simulink model "simulink_model_traverse"  (R2021b)
settings: Solver=ode45  StartTime=0.0  StopTime=20  RelTol=1e-3
model workspace (MAT data in the model file):
  real_gyro_traverse_system = frd
  real_gyro_traverse_system.IOSize_ = [1 1]
  real_gyro_traverse_system.Data_ = ltipack.frddata
  real_gyro_traverse_system.Data_.Frequency = [6.28310441366 6.33210341522 6.38148441394 6.43125040589 6.48140513613 6.53195010269 6.58288979967 6.63422647409 6.68596387104 6.73810423754 6.7906520677 6.84360885953 ... (801 elements, 801x1)]
  real_gyro_traverse_system.Data_.Response = [0.0415989533067-0.25452619791i 0.0397742167115-0.252204239368i 0.0379806235433-0.249895423651i 0.0362177714705-0.247599869967i 0.0344851389527-0.245317786932i 0.0297197960317-0.238508492708i 0.0252005718648-0.231830269098i 0.0209181196988-0.225282818079i 0.0168635360897-0.218866020441i 0.0203672014177-0.220373362303i 0.0239223502576-0.221838980913i 0.0275287441909-0.223261684179i ... (801 elements, 1x1x801)]
  real_gyro_traverse_system.Data_.Delay.Input = 0
  real_gyro_traverse_system.Data_.Delay.Output = 0
  real_gyro_traverse_system.Data_.Delay.IO = 0
  real_gyro_traverse_system.Data_.Ts = 0
  real_gyro_traverse_system.FrequencyUnit_ = 'Hz'
values from neighbouring files (symbols this model uses):
  fric_gear_motor_traverse = 0.021    [loading_project.m]
  fric_gear_turrent_gun_traverse = 1.272    [loading_project.m]
  ts3 = 10^-3    (= 0.001)    [loading_project.m]
libraries: simulink x3, dspsrcs4 x1
(part 1 of 2)
settings Model: Creator=itama  LastModifiedBy=noait

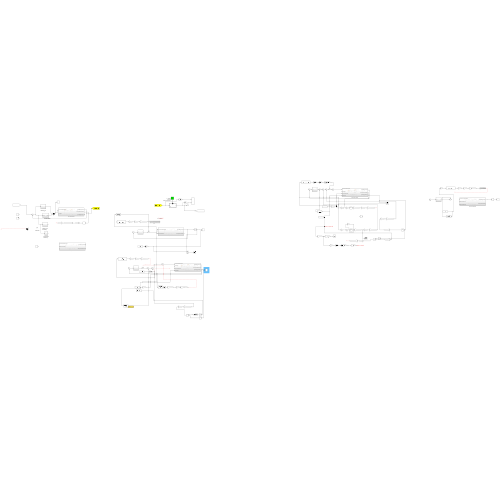
[thumbnail: Simulink's stored preview of the top-level diagram]
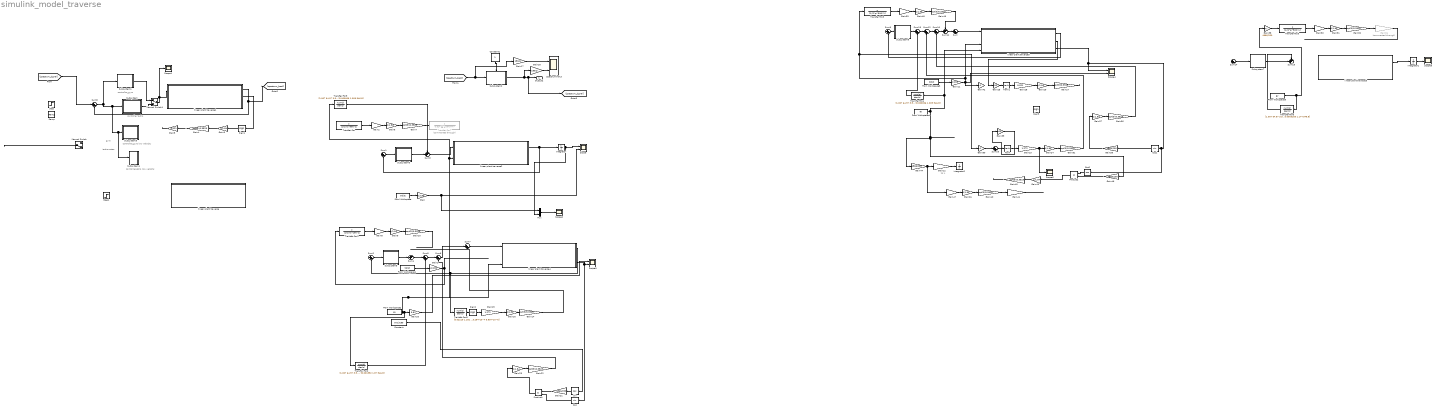
== system simulink_model_traverse ==
  note: controller_gyro
  note: gyro
  note: tachometer
  note: controller tacho
  note: controller_gyro
      | low velocity
  note: controller_taho
      | low velocity
  note: 1/J L
  note: 1/J L
  Constant : Constant  Value=0*pi/180  SampleTime=-1
  Constant1 : Constant  OutDataTypeStr=boolean
      settings: AttributesFormatString=1 - START\n0 -STOP\ninternal spectrum
      settings: OpenFcn=|
      | if get_param(gcbh,'value')-48 set_param(gcbh,'value','0','backgroundcolor','red');
      | else set_param(gcbh,'value','1','backgroundcolor','green');
      | end
  Cos : Trigonometry
  Cos1 : Trigonometry
  Cos2 : Trigonometry  Operator=cos
  From Workspace : FromWorkspace  VariableName=trdist  SampleTime=ts3/3  ZeroCross=off  OutputAfterFinalValue=Setting to zero
  From Workspace1 : FromWorkspace  VariableName=trdist  SampleTime=ts3/3  ZeroCross=off  OutputAfterFinalValue=Setting to zero
  From Workspace2 : FromWorkspace  VariableName=gy  SampleTime=ts3/3  Interpolate=off  ZeroCross=off  OutputAfterFinalValue=Setting to zero
  From Workspace3 : FromWorkspace  VariableName=trdist  SampleTime=ts3/3  Interpolate=off  ZeroCross=off  OutputAfterFinalValue=Setting to zero
  From Workspace4 : FromWorkspace  VariableName=gy  SampleTime=ts3/3  Interpolate=off  ZeroCross=off  OutputAfterFinalValue=Setting to zero
  From Workspace5 : FromWorkspace  VariableName=gy  SampleTime=ts3/3  Interpolate=off  ZeroCross=off  OutputAfterFinalValue=Setting to zero
  Gain : Gain  Gain=pi/180
  Gain1 : Gain  Gain=pi/180
  Gain{4,7,10,14,22,27,32,36,40,45,49,51} (12 alike) : Gain  Gain=sqrt(3)/0.3525
  Gain11 : Gain  Gain=pi/180
  Gain12 : Gain  Gain=-1/0.2189801
  Gain13 : Gain  Gain=1.272
  Gain15 : Gain  Gain=1.272
  Gain{3,6,9,16,23..24,26,29,31,37,43,48} (12 alike) : Gain  Gain=1/1.84
  Gain17 : Gain  Gain=180/pi
  Gain18 : Gain  Gain=180/pi
  Gain{2,8,30,33,47} (5 alike) : Gain  Gain=0.0093
  Gain20 : Gain  Gain=9.81
  Gain{21,35,38,44,46} (5 alike) : Gain  Gain=4866/200
  Gain25 : Gain  Gain=100
  Gain28 : Gain  Gain=0.021
  Gain34 : Gain  Commented=through  Gain=1/0.2189801
  Gain39 : Gain  Gain=100
  Gain41 : Gain  Gain=1/0.2189801
  Gain42 : Gain  Gain=-1
  Gain5 : Gain  Gain=0.021
  Gain50 : Gain  Gain=-1
  Integrator : Integrator
  Integrator1 : Integrator
  Integrator2 : Integrator  ZeroCross=off
  Manual Switch : ManualSwitch  CurrentSetting=0
  Manual Switch1 : ManualSwitch
  Mux : Mux  Inputs=2
  Product1 : Product
  Product2 : Product
  Ramp : simulink/Sources/Ramp  slope=1  start=0  InitialOutput=0
  Scope : Scope  NumInputPorts=2
  Scope{1..2,5..6} (4 alike) : Scope
  Scope3 : Scope  NumInputPorts=2
  Scope4 : Scope  NumInputPorts=2
  Sign1 : Signum
  Sign2 : Signum
  Sign3 : Signum  ZeroCross=off
  Sin : Trigonometry  Operator=cos
  SpectrumInOut : Scope  NumInputPorts=2
  Step : Step  After=0.05  SampleTime=0
  Step1 : Step  After=10*pi/180  SampleTime=0
  Subsystem : Subsystem
  Subsystem1 : Subsystem
  Subsystem2 : Subsystem  mask{GAIN=1%2*pi/180%0.5*pi/180, InitFreq=1, TargetTime=500, FreqAtTime=500}
      mask prompts: InitFreq "INITIAL FREQUENCY"; TargetTime "Target Time"; FreqAtTime "Frequency at Time"
  Subsystem3 : Subsystem
  Subsystem4 : Subsystem
  Subsystem5 : Subsystem
  Subsystem6 : Subsystem
  Subsystem7 : Subsystem
  Subsystem8 : Subsystem
  Sum{,5,7,12..13,16} (6 alike) : Sum  Inputs=|++
  Sum{1..2,6,8..10,14} (7 alike) : Sum  Inputs=|+-
  Sum11 : Sum  Inputs=-+|
  Sum15 : Sum  Inputs=++|
  Sum3 : Sum  Inputs=++|
  Sum4 : Sum  Inputs=-+|
  Tanh : Trigonometry  Operator=tanh
  Tanh1 : Trigonometry  Operator=tanh
  Transfer Fcn : TransferFcn  Numerator=[1 0]  Denominator=[1/(2*pi*500) 1]
  Transfer Fcn1 : TransferFcn  Numerator=[1 0]  Denominator=[1/(2*pi*100) 1]
  Transfer Fcn2 : TransferFcn  Numerator=[1.007 64.97 3.552*10^4]  Denominator=[0.001592 1.87 546.8]
  Transfer Fcn3 : TransferFcn  Numerator=[1 0]  Denominator=[1/(2*pi*500) 1]
  Transfer Fcn4 : TransferFcn  Numerator=[1.007 64.97 3.552*10^4]  Denominator=[0.000006 1.009 546.8]
  Transfer Fcn5 : TransferFcn  Numerator=[1 0]  Denominator=[1/(2*pi*500) 1]
  Transfer Fcn6 : TransferFcn  Numerator=[1.007 64.97 3.552*10^4]  Denominator=[0.0003183 1.174 546.8]
  Transfer Fcn7 : TransferFcn  Commented=through  Numerator=[1 0]  Denominator=[0.6 328.0575777]
  Transfer Fcn8 : TransferFcn  Numerator=[0.02219 1.182 1026 1.42*10^4 5.857*10^6]  Denominator="[0.003183 2.538  528.2 3.284*10^4 5.857*10^6]"
  Transfer Fcn9 : TransferFcn  Numerator=[1.007 64.97 3.552*10^4]  Denominator=[0.000006 1.009 546.8]
  linear plant traverse : Subsystem
  linear plant traverse1 : Subsystem
  linear plant traverse2 : Subsystem
  linear plant traverse3 : Subsystem
  linear plant traverse4 : Subsystem
  linear plant traverse5 : Subsystem
  Output2 : Outport
  wires:
  Manual Switch/1 -> ?
  Subsystem/1(Out1) -> Manual Switch1/2
  Constant1/1 -> Subsystem2/Enable
  Subsystem2/1(Output2) -> [spectrum_signal], Output2/1, Gain18/1
  Gain18/1 -> SpectrumInOut/2
  [spectrum_back] -> Gain17/1, Subsystem2/1(Input)
  Gain17/1 -> SpectrumInOut/1
  Sum8/1 -> Subsystem1/1(In1), Subsystem4/1(In1), Subsystem3/1(In1), Subsystem/1(In1)
  Manual Switch1/1 -> Scope1/1, linear plant traverse1/1(current command traverse)
  linear plant traverse1/2(motor speed tachometer) -> Sign1/1
  Gain4/1 -> Gain5/1
  Gain3/1 -> Gain4/1
  Sign1/1 -> Gain3/1
  Subsystem1/1(Output) -> Manual Switch1/1
  Gain5/1 -> ?
  linear plant traverse1/1(gun speed gyroscope) -> [spectrum_back], Sum8/2
  Sum1/1 -> Subsystem6/1(In1)
  linear plant traverse2/1(gun speed gyroscope) -> Integrator/1, Sum1/2
  From Workspace/1 -> Gain/1
  Gain/1 -> Scope/2, Mux/1
  Integrator/1 -> Mux/2, Scope/1
  Mux/1 -> Scope2/1
  From Workspace1/1 -> Gain1/1
  Gain1/1 -> Transfer Fcn1/1
  Sum2/1 -> Subsystem5/1(In1)
  Subsystem6/1(Output) -> Sum3/2
  Gain2/1 -> Gain6/1
  Gain6/1 -> Gain7/1
  Transfer Fcn/1 -> Gain2/1
  Sum3/1 -> linear plant traverse2/1(current command traverse)
  Subsystem5/1(Output) -> Sum4/2
  Gain9/1 -> Gain10/1
  Gain8/1 -> Gain9/1
  Gain10/1 -> ?
  linear plant traverse4/1(gun speed gyroscope) -> Transfer Fcn8/1, Sum2/2
  Sum4/1 -> Sum5/1
  Sum5/1 -> Sum6/1
  Gain16/1 -> Gain14/1
  Gain15/1 -> Gain16/1
  Sign2/1 -> Gain15/1
  Constant/1 -> Sin/1
  linear plant traverse4/3("gun angle gyroscope ") -> Cos/1, Scope3/2
  Sum6/1 -> Sum7/1
  Gain21/1 -> Product1/1
  Sin/1 -> Gain21/1
  Cos/1 -> Product1/2
  Sum7/1 -> linear plant traverse4/1(current command traverse)
  Gain23/1 -> Gain22/1
  Product1/1 -> Gain23/1
  Gain14/1 -> ?
  Transfer Fcn1/1 -> Gain8/1
  Gain22/1 -> Sum6/2
  Gain20/1 -> Scope3/1
  [spectrum_signal] -> Sum8/1
  Transfer Fcn2/1 -> Sum5/2
  Transfer Fcn8/1 -> Sign2/1
  Transfer Fcn4/1 -> Sum13/2
  Gain43/1 -> Gain45/1
  Gain39/1 -> Tanh/1
  From Workspace5/1 -> Transfer Fcn6/1, Gain38/1
  Gain44/1 -> Gain47/1, Gain12/1
  From Workspace4/1 -> Gain46/1, Gain44/1, linear plant traverse5/4(acceleration), Transfer Fcn4/1
  Integrator1/1 -> Scope5/1
  Tanh/1 -> Gain13/1
  Product2/1 -> Gain43/1
  Gain50/1 -> Sum16/1
  Gain32/1 -> Gain34/1
  Sum12/1 -> Sum10/1
  Gain48/1 -> Gain49/1
  Cos2/1 -> Product2/1
  linear plant traverse5/2(motor speed tachometer) -> Gain25/1
  Subsystem8/1(Output) -> Sum13/1
  Transfer Fcn5/1 -> Gain30/1
  Gain30/1 -> Gain31/1
  Gain31/1 -> Gain32/1
  Subsystem7/1(Output) -> Sum15/2
  Transfer Fcn6/1 -> Sum15/1
  Gain36/1 -> Sum10/2
  Sum16/1 -> Gain39/1
  Gain40/1 -> Gain41/1
  Gain26/1 -> Gain40/1
  Sum9/1 -> Subsystem8/1(In1)
  Gain33/1 -> Gain48/1
  From Workspace3/1 -> Gain11/1
  Gain28/1 -> Gain29/1
  linear plant traverse5/3("gun angle gyroscope ") -> Cos2/1, Cos1/1, Scope4/1
  Cos1/1 -> Gain35/1
  Gain49/1 -> Sum11/1
  Gain29/1 -> Gain27/1
  Sum10/1 -> Sum11/2
  Gain11/1 -> Gain42/1, linear plant traverse5/3(external distribution), Transfer Fcn3/1, Gain50/1, Scope4/2
  Gain37/1 -> Gain36/1
  Gain38/1 -> Transfer Fcn5/1
  linear plant traverse5/1(gun speed gyroscope) -> Sum9/2
  Gain45/1 -> ?
  Gain51/1 -> Sum12/2
  Sum/1 -> linear plant traverse5/1(current command traverse)
  Gain13/1 -> Scope6/1, Gain24/1
  Tanh1/1 -> Gain28/1
  Transfer Fcn3/1 -> Gain33/1
  linear plant traverse3/1(gun speed gyroscope) -> Integrator1/1
  Sum14/1 -> Subsystem7/1(In1)
  Gain24/1 -> Gain51/1
  Gain12/1 -> Integrator2/1
  Gain35/1 -> Gain37/1
  Sum13/1 -> Sum12/1
  Gain46/1 -> Product2/2
  Gain47/1 -> Gain26/1
  Sum11/1 -> Sum/1
  Gain27/1 -> ?
  Gain34/1 -> ?
  Gain25/1 -> Tanh1/1
  Gain41/1 -> ?
  Gain7/1 -> Transfer Fcn7/1
  ? -> ?  "velocity_feedback"
  From Workspace2/1 -> Transfer Fcn9/1, linear plant traverse2/2(external distribution), linear plant traverse4/4(acceleration), Transfer Fcn2/1, Gain20/1
  Transfer Fcn9/1 -> Sum3/1

== system simulink_model_traverse/Subsystem ==
  note: notch_filter
  note: inverse model motor-load
  note: phase lead
  note: cancel zero from tachomete
  In1 : Inport
  Add2 : Sum
  Gain10 : Gain  Gain=2*pi*3
  Gain9 : Gain  Gain=25.6
  Integrator4 : Integrator
  Transfer Fcn : TransferFcn  Numerator=[1/(2*pi*4.5)^2 0.014/1.7 1]  Denominator=[1/(2*pi*3.62)^2 0.014/1.7 1]
  Transfer Fcn1 : TransferFcn  Denominator=[1/(2*pi*6.06)^2 0.6/328.057 1]
  Transfer Fcn4 : TransferFcn  Numerator=[0.0083 1]  Denominator=[0.0011 1]
  Transfer Fcn5 : TransferFcn  Numerator=[1 2*0.08*2*36.1*pi (2*pi*36.1)^2]  Denominator=[1 2*0.94*2*36.1*pi (2*pi*36.1)^2]
  Out1 : Outport
  wires:
  Add2/1 -> Transfer Fcn/1
  Integrator4/1 -> Add2/1
  Gain9/1 -> Gain10/1, Add2/2
  Gain10/1 -> Integrator4/1
  In1/1 -> Gain9/1  "current"
  Transfer Fcn5/1 -> Out1/1  "c_output"
  Transfer Fcn1/1 -> Transfer Fcn4/1
  Transfer Fcn/1 -> Transfer Fcn1/1
  Transfer Fcn4/1 -> Transfer Fcn5/1

== system simulink_model_traverse/Subsystem1 ==
  note: anti_notch
  note: notch_filter
  note: notch_filter
  note: notch_filter
  In1 : Inport
  Add3 : Sum  Inputs=+++
  Gain : Gain  Gain=0.0118
  Gain1 : Gain  Gain=26
  Gain11 : Gain  Gain=2*pi*1.4
  Gain12 : Gain  Gain=24
  Integrator5 : Integrator
  Transfer Fcn : TransferFcn  Numerator=[1 0]  Denominator=[1/(2*pi*100) 1]
  Transfer Fcn1 : TransferFcn  Numerator=[1 2*0.08*2*68*pi (2*pi*68)^2]  Denominator=[1 2*0.94*2*68*pi (2*pi*68)^2]
  Transfer Fcn2 : TransferFcn  Numerator=[1 2*0.5*2*18*pi (2*pi*18)^2]  Denominator=[1 2*0.05*2*18*pi (2*pi*18)^2]
  Transfer Fcn3 : TransferFcn  Numerator=[1 2*0.08*2*450*pi (2*pi*450)^2]  Denominator=[1 2*0.94*2*450*pi (2*pi*450)^2]
  Transfer Fcn4 : TransferFcn  Numerator=[1 2*0.05*2*13*pi (2*pi*13)^2]  Denominator=[1 2*0.65*2*13*pi (2*pi*13)^2]
  Transfer Fcn6 : TransferFcn  Numerator=[1 2*0.08*2*30*pi (2*pi*30)^2]  Denominator=[1 2*0.94*2*30*pi (2*pi*30)^2]
  Output : Outport
  wires:
  Gain11/1 -> Integrator5/1
  Integrator5/1 -> Add3/1
  Transfer Fcn4/1 -> Transfer Fcn6/1
  Transfer Fcn2/1 -> Transfer Fcn4/1
  Gain/1 -> Transfer Fcn/1
  Transfer Fcn/1 -> Add3/3
  Transfer Fcn6/1 -> Transfer Fcn1/1
  Add3/1 -> Transfer Fcn2/1
  Gain12/1 -> Gain/1
  Gain1/1 -> Gain11/1, Add3/2
  In1/1 -> Gain12/1, Gain1/1
  Transfer Fcn1/1 -> Transfer Fcn3/1
  Transfer Fcn3/1 -> Output/1

== system simulink_model_traverse/Subsystem2 ==
  Input : Inport
  Enable : EnablePort  StatesWhenEnabling=reset
  Chirp : dspsrcs4/Chirp  sweep=Linear  mode=Unidirectional  f0=1  f1=160  t1=160  Tsweep=160  phase=0  Ts=1/1000  spf=1  datatype=Double  OutputFrames=off
  Chirp Signal : simulink/Sources/Chirp Signal  Commented=on  f1=InitFreq  T=TargetTime  f2=FreqAtTime
  Chirp Signal1 : simulink/Sources/Chirp Signal  f1=1  T=160  f2=160
  Mux2 : Mux  Inputs=2
  Scope2 : Scope
  TSABAD_out_log : Scope
  gain 3 : Gain  Gain=GAIN  SaturateOnIntegerOverflow=on  SampleTime=ts3  OutDataTypeStr=Inherit: Same as input  ParamDataTypeStr=Inherit: Same as input
  Output2 : Outport
  wires:
  gain 3/1 -> Output2/1, Mux2/1
  Chirp Signal/1 -> ?
  Input/1 -> Mux2/2
  Mux2/1 -> TSABAD_out_log/1
  Chirp Signal1/1 -> gain 3/1, Scope2/1

== system simulink_model_traverse/Subsystem3 ==
  note: anti_notch
  note: notch_filter
  note: notch_filter
  note: notch_filter
  In1 : Inport
  Add3 : Sum
  Gain1 : Gain  Gain=26
  Gain11 : Gain  Gain=2*pi*2.5
  Integrator5 : Integrator
  Transfer Fcn1 : TransferFcn  Numerator=[1 2*0.08*2*68*pi (2*pi*68)^2]  Denominator=[1 2*0.94*2*68*pi (2*pi*68)^2]
  Transfer Fcn2 : TransferFcn  Numerator=[1 2*0.5*2*18*pi (2*pi*18)^2]  Denominator=[1 2*0.05*2*18*pi (2*pi*18)^2]
  Transfer Fcn3 : TransferFcn  Numerator=[1 2*0.08*2*450*pi (2*pi*450)^2]  Denominator=[1 2*0.94*2*450*pi (2*pi*450)^2]
  Transfer Fcn4 : TransferFcn  Numerator=[1 2*0.05*2*13*pi (2*pi*13)^2]  Denominator=[1 2*0.65*2*13*pi (2*pi*13)^2]
  Transfer Fcn6 : TransferFcn  Numerator=[1 2*0.08*2*30*pi (2*pi*30)^2]  Denominator=[1 2*0.94*2*30*pi (2*pi*30)^2]
  Output : Outport
  wires:
  Gain11/1 -> Integrator5/1
  Integrator5/1 -> Add3/1
  Transfer Fcn4/1 -> Transfer Fcn6/1
  Transfer Fcn2/1 -> Transfer Fcn4/1
  Transfer Fcn6/1 -> Transfer Fcn1/1
  Add3/1 -> Transfer Fcn2/1
  Gain1/1 -> Gain11/1, Add3/2
  In1/1 -> Gain1/1
  Transfer Fcn1/1 -> Transfer Fcn3/1
  Transfer Fcn3/1 -> Output/1

== system simulink_model_traverse/Subsystem4 ==
  In1 : Inport
  Gain : Gain  Gain=2*pi*1000
  Gain1 : Gain  Gain=10
  Sum : Sum  Inputs=|++
  Transfer Fcn : TransferFcn  Denominator="[1  0]"
  Out1 : Outport
  wires:
  Sum/1 -> Out1/1
  Gain1/1 -> Sum/2
  Gain/1 -> Transfer Fcn/1
  Transfer Fcn/1 -> Sum/1
  In1/1 -> Gain1/1, Gain/1

== system simulink_model_traverse/Subsystem5 ==
  note: anti_notch
  note: notch_filter
  note: notch_filter
  note: notch_filter
  In1 : Inport
  Add3 : Sum  Inputs=+++
  Gain : Gain  Gain=0.0118
  Gain1 : Gain  Gain=26
  Gain11 : Gain  Gain=2*pi*1.4
  Gain12 : Gain  Gain=24
  Integrator5 : Integrator
  Transfer Fcn : TransferFcn  Numerator=[1 0]  Denominator=[1/(2*pi*100) 1]
  Transfer Fcn1 : TransferFcn  Numerator=[1 2*0.08*2*68*pi (2*pi*68)^2]  Denominator=[1 2*0.94*2*68*pi (2*pi*68)^2]
  Transfer Fcn2 : TransferFcn  Numerator=[1 2*0.5*2*18*pi (2*pi*18)^2]  Denominator=[1 2*0.05*2*18*pi (2*pi*18)^2]
  Transfer Fcn3 : TransferFcn  Numerator=[1 2*0.08*2*450*pi (2*pi*450)^2]  Denominator=[1 2*0.94*2*450*pi (2*pi*450)^2]
  Transfer Fcn4 : TransferFcn  Numerator=[1 2*0.05*2*13*pi (2*pi*13)^2]  Denominator=[1 2*0.65*2*13*pi (2*pi*13)^2]
  Transfer Fcn6 : TransferFcn  Numerator=[1 2*0.08*2*30*pi (2*pi*30)^2]  Denominator=[1 2*0.94*2*30*pi (2*pi*30)^2]
  Output : Outport
  wires:
  Gain11/1 -> Integrator5/1
  Integrator5/1 -> Add3/1
  Transfer Fcn4/1 -> Transfer Fcn6/1
  Transfer Fcn2/1 -> Transfer Fcn4/1
  Gain/1 -> Transfer Fcn/1
  Transfer Fcn/1 -> Add3/3
  Transfer Fcn6/1 -> Transfer Fcn1/1
  Add3/1 -> Transfer Fcn2/1
  Gain12/1 -> Gain/1
  Gain1/1 -> Gain11/1, Add3/2
  In1/1 -> Gain12/1, Gain1/1
  Transfer Fcn1/1 -> Transfer Fcn3/1
  Transfer Fcn3/1 -> Output/1

== system simulink_model_traverse/Subsystem6 ==
  note: anti_notch
  note: notch_filter
  note: notch_filter
  note: notch_filter
  In1 : Inport
  Add3 : Sum  Inputs=+++
  Gain : Gain  Gain=0.0118
  Gain1 : Gain  Gain=26
  Gain11 : Gain  Gain=2*pi*1.4
  Gain12 : Gain  Gain=24
  Integrator5 : Integrator
  Transfer Fcn : TransferFcn  Numerator=[1 0]  Denominator=[1/(2*pi*100) 1]
  Transfer Fcn1 : TransferFcn  Numerator=[1 2*0.08*2*68*pi (2*pi*68)^2]  Denominator=[1 2*0.94*2*68*pi (2*pi*68)^2]
  Transfer Fcn2 : TransferFcn  Numerator=[1 2*0.5*2*18*pi (2*pi*18)^2]  Denominator=[1 2*0.05*2*18*pi (2*pi*18)^2]
  Transfer Fcn3 : TransferFcn  Numerator=[1 2*0.08*2*450*pi (2*pi*450)^2]  Denominator=[1 2*0.94*2*450*pi (2*pi*450)^2]
  Transfer Fcn4 : TransferFcn  Numerator=[1 2*0.05*2*13*pi (2*pi*13)^2]  Denominator=[1 2*0.65*2*13*pi (2*pi*13)^2]
  Transfer Fcn6 : TransferFcn  Numerator=[1 2*0.08*2*30*pi (2*pi*30)^2]  Denominator=[1 2*0.94*2*30*pi (2*pi*30)^2]
  Output : Outport
  wires:
  Gain11/1 -> Integrator5/1
  Integrator5/1 -> Add3/1
  Transfer Fcn4/1 -> Transfer Fcn6/1
  Transfer Fcn2/1 -> Transfer Fcn4/1
  Gain/1 -> Transfer Fcn/1
  Transfer Fcn/1 -> Add3/3
  Transfer Fcn6/1 -> Transfer Fcn1/1
  Add3/1 -> Transfer Fcn2/1
  Gain12/1 -> Gain/1
  Gain1/1 -> Gain11/1, Add3/2
  In1/1 -> Gain12/1, Gain1/1
  Transfer Fcn1/1 -> Transfer Fcn3/1
  Transfer Fcn3/1 -> Output/1

== system simulink_model_traverse/Subsystem7 ==
  note: anti_notch
  note: notch_filter
  note: notch_filter
  note: notch_filter
  In1 : Inport
  Add3 : Sum  Inputs=+++
  Gain : Gain  Gain=0.0118
  Gain1 : Gain  Gain=26
  Gain11 : Gain  Gain=2*pi*1.4
  Gain12 : Gain  Gain=24
  Integrator5 : Integrator
  Transfer Fcn : TransferFcn  Numerator=[1 0]  Denominator=[1/(2*pi*500) 1]
  Transfer Fcn1 : TransferFcn  Numerator=[1 2*0.08*2*68*pi (2*pi*68)^2]  Denominator=[1 2*0.94*2*68*pi (2*pi*68)^2]
  Transfer Fcn2 : TransferFcn  Numerator=[1 2*0.5*2*18*pi (2*pi*18)^2]  Denominator=[1 2*0.05*2*18*pi (2*pi*18)^2]
  Transfer Fcn3 : TransferFcn  Numerator=[1 2*0.08*2*450*pi (2*pi*450)^2]  Denominator=[1 2*0.94*2*450*pi (2*pi*450)^2]
  Transfer Fcn4 : TransferFcn  Numerator=[1 2*0.05*2*13*pi (2*pi*13)^2]  Denominator=[1 2*0.65*2*13*pi (2*pi*13)^2]
  Transfer Fcn6 : TransferFcn  Numerator=[1 2*0.08*2*30*pi (2*pi*30)^2]  Denominator=[1 2*0.94*2*30*pi (2*pi*30)^2]
  Output : Outport
  wires:
  Gain11/1 -> Integrator5/1
  Integrator5/1 -> Add3/1
  Transfer Fcn4/1 -> Transfer Fcn6/1
  Transfer Fcn2/1 -> Transfer Fcn4/1
  Gain/1 -> Transfer Fcn/1
  Transfer Fcn/1 -> Add3/3
  Transfer Fcn6/1 -> Transfer Fcn1/1
  Add3/1 -> Transfer Fcn2/1
  Gain12/1 -> Gain/1
  Gain1/1 -> Gain11/1, Add3/2
  In1/1 -> Gain12/1, Gain1/1
  Transfer Fcn1/1 -> Transfer Fcn3/1
  Transfer Fcn3/1 -> Output/1

== system simulink_model_traverse/Subsystem8 ==
  note: anti_notch
  note: notch_filter
  note: notch_filter
  note: notch_filter
  In1 : Inport
  Add3 : Sum  Inputs=+++
  Gain : Gain  Gain=0.0118
  Gain1 : Gain  Gain=26
  Gain11 : Gain  Gain=2*pi*1.4
  Gain12 : Gain  Gain=24
  Integrator5 : Integrator
  Transfer Fcn : TransferFcn  Numerator=[1 0]  Denominator=[1/(2*pi*500) 1]
  Transfer Fcn1 : TransferFcn  Numerator=[1 2*0.08*2*68*pi (2*pi*68)^2]  Denominator=[1 2*0.94*2*68*pi (2*pi*68)^2]
  Transfer Fcn2 : TransferFcn  Numerator=[1 2*0.5*2*18*pi (2*pi*18)^2]  Denominator=[1 2*0.05*2*18*pi (2*pi*18)^2]
  Transfer Fcn3 : TransferFcn  Numerator=[1 2*0.08*2*450*pi (2*pi*450)^2]  Denominator=[1 2*0.94*2*450*pi (2*pi*450)^2]
  Transfer Fcn4 : TransferFcn  Numerator=[1 2*0.05*2*13*pi (2*pi*13)^2]  Denominator=[1 2*0.65*2*13*pi (2*pi*13)^2]
  Transfer Fcn6 : TransferFcn  Numerator=[1 2*0.08*2*30*pi (2*pi*30)^2]  Denominator=[1 2*0.94*2*30*pi (2*pi*30)^2]
  Output : Outport
  wires:
  Gain11/1 -> Integrator5/1
  Integrator5/1 -> Add3/1
  Transfer Fcn4/1 -> Transfer Fcn6/1
  Transfer Fcn2/1 -> Transfer Fcn4/1
  Gain/1 -> Transfer Fcn/1
  Transfer Fcn/1 -> ?
  Transfer Fcn6/1 -> Transfer Fcn1/1
  Add3/1 -> Transfer Fcn2/1
  Gain12/1 -> Gain/1
  Gain1/1 -> Gain11/1, Add3/2
  In1/1 -> Gain12/1, Gain1/1
  Transfer Fcn1/1 -> Transfer Fcn3/1
  Transfer Fcn3/1 -> Output/1

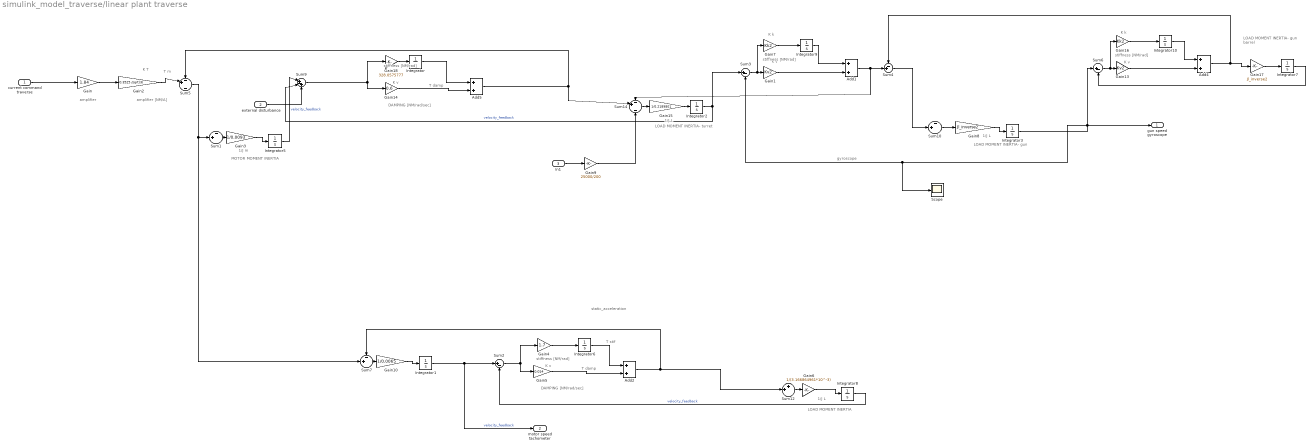
== system simulink_model_traverse/linear plant traverse ==
  note: gyroscope
  note: K v
  note: T m
  note: stiffness
      | [NM/rad]
  note: K T
  note: K k
  note: MOTOR
      | MOMENT INERTIA
  note: amplifier
      | [NM/A]
  note: 1/J m
  note: K v
  note: stiffness
      | [NM/rad]
  note: K k
  note: static_acceleration
  note: LOAD
      | MOMENT INERTIA- gun
  note: 1/J L
  note: 1/J L
  note: stiffness
      | [NM/rad]
  note: T damp
  note: DAMPING
      | [NM/rad/sec]
  note: LOAD
      | MOMENT INERTIA
  note: K v
  note: T stif
  note: stiffness
      | [NM/rad]
  note: T damp
  note: DAMPING
      | [NM/rad/sec]
  note: LOAD
      | MOMENT INERTIA- turret
  note: K v
  note: 1/J L
  note: LOAD
      | MOMENT INERTIA- gun barrel
  note: amplifier
  current command traverse : Inport
  external disturbance : Inport  Port=2
  In1 : Inport  Port=3
  Add{1..2,4..5} (4 alike) : Sum
  Gain : Gain  Gain=1.84
  Gain1 : Gain  Gain=Kv2  mask{Kv2=0.1645}
      mask prompts: Kv2 "damping2"
  Gain10 : Gain  Gain=1/0.0065
  Gain13 : Gain  Gain=Kv2  mask{Kv2=0.015}
      mask prompts: Kv2 "damping2"
  Gain14 : Gain  Gain=0.6
  Gain15 : Gain  Gain=1/0.2189801
  Gain16 : Gain  Gain=Kk2  mask{Kk2=44.63119054}
      mask prompts: Kk2 "stifnes_2"
  Gain17 : Gain  Gain=Jl_inverse2  mask{Jl_inverse2=1/(3.649668334*10^-3)}
      mask prompts: Jl_inverse2 "inverse_moment_inertia2"
  Gain18 : Gain  Gain=328.0575777
  Gain2 : Gain  Gain=0.3525 /sqrt(3)
  Gain3 : Gain  Gain=1/0.0093
  Gain4 : Gain  Gain=1.7
  Gain5 : Gain  Gain=0.014
  Gain6 : Gain  Gain=1/(3.166864961*10^-3)
  Gain7 : Gain  Gain=Kk2  mask{Kk2=78.78413144}
      mask prompts: Kk2 "stifnes_2"
  Gain8 : Gain  Gain=Jl_inverse2  mask{Jl_inverse2=1/(3.649668334*10^-3)}
      mask prompts: Jl_inverse2 "inverse_moment_inertia2"
  Gain9 : Gain  Gain=25000/200
  Integrator{,6..7,9..10} (5 alike) : Integrator
  Integrator{1..3,5,8} (5 alike) : Integrator  ZeroCross=off
  Scope : Scope
  Sum1 : Sum  Inputs=-+|  SaturateOnIntegerOverflow=on
  Sum10 : Sum  Inputs=-+|  SaturateOnIntegerOverflow=on
  Sum12 : Sum  Inputs=++|  SaturateOnIntegerOverflow=on
  Sum14 : Sum  Inputs=-+|-  SaturateOnIntegerOverflow=on
  Sum2 : Sum  Inputs=|+-
  Sum3 : Sum  Inputs=|+-
  Sum4 : Sum  Inputs=-+|
  Sum5 : Sum  Inputs=-+|-
  Sum6 : Sum  Inputs=|+-
  Sum7 : Sum  Inputs=-+|  SaturateOnIntegerOverflow=on
  Sum9 : Sum  Inputs=|+-+
  gun speed gyroscope : Outport
  motor speed tachometer : Outport  Port=2
  wires:
  Gain16/1 -> Integrator10/1
  Sum5/1 -> Sum7/2, Sum1/2
  Integrator7/1 -> Sum6/2
  Gain/1 -> Gain2/1
  Integrator9/1 -> Add1/1
  Gain18/1 -> Integrator/1
  Gain3/1 -> Integrator5/1
  Gain13/1 -> Add4/2
  Add1/1 -> Sum14/1, Sum4/2
  Gain6/1 -> Integrator8/1
  Gain14/1 -> Add5/2
  Gain2/1 -> Sum5/2
  Integrator/1 -> Add5/1
  Sum3/1 -> Gain7/1, Gain1/1
  Gain1/1 -> Add1/2
  Gain10/1 -> Integrator1/1
  Gain17/1 -> Integrator7/1
  Gain7/1 -> Integrator9/1
  Integrator8/1 -> Sum2/2  "velocity_feedback"
  Integrator3/1 -> gun speed gyroscope/1, Scope/1, Sum3/2, Sum6/1
  Sum2/1 -> Gain5/1, Gain4/1
  Sum10/1 -> Gain8/1
  Add4/1 -> Sum4/1, Gain17/1
  Integrator10/1 -> Add4/1
  Add2/1 -> Sum7/1, Sum12/2
  Integrator6/1 -> Add2/1
  Sum4/1 -> Sum10/2
  Integrator2/1 -> Sum3/1, Sum9/2  "velocity_feedback"
  Sum9/1 -> Gain18/1, Gain14/1
  Sum6/1 -> Gain16/1, Gain13/1
  Sum14/1 -> Gain15/1
  Gain15/1 -> Integrator2/1
  Gain5/1 -> Add2/2
  Sum7/1 -> Gain10/1
  Sum12/1 -> Gain6/1
  Sum1/1 -> Gain3/1
  Integrator5/1 -> Sum9/1  "velocity_feedback"
  Add5/1 -> Sum14/2, Sum5/1
  Gain4/1 -> Integrator6/1
  Gain8/1 -> Integrator3/1
  Integrator1/1 -> motor speed tachometer/1, Sum2/1  "velocity_feedback"
  current command traverse/1 -> Gain/1
  external disturbance/1 -> Sum9/3
  In1/1 -> Gain9/1
  Gain9/1 -> Sum14/3

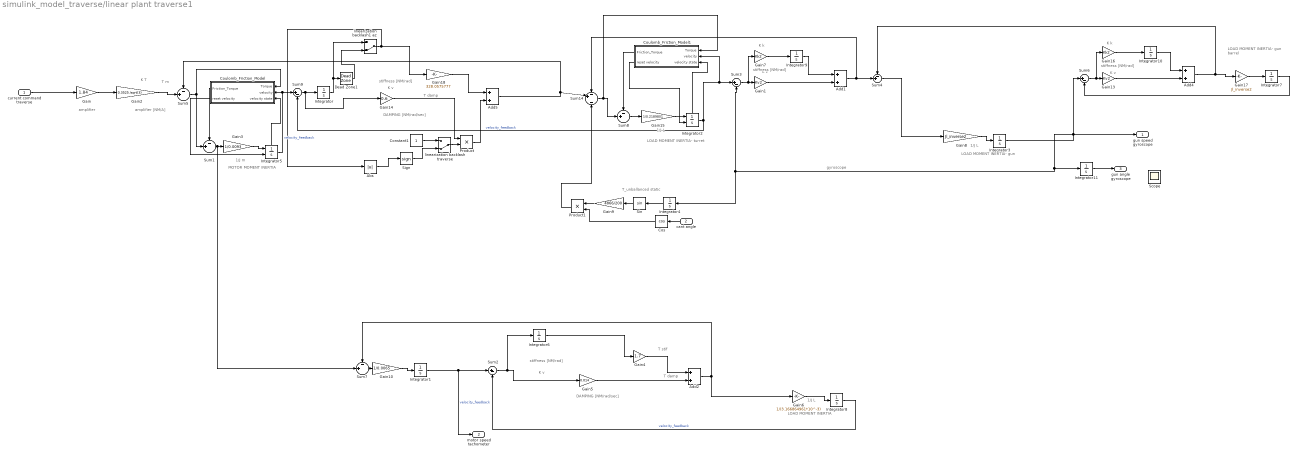
== system simulink_model_traverse/linear plant traverse1 ==
  note: gyroscope
  note: T_unballanced static
  note: K v
  note: T m
  note: stiffness
      | [NM/rad]
  note: K T
  note: K k
  note: MOTOR
      | MOMENT INERTIA
  note: amplifier
      | [NM/A]
  note: 1/J m
  note: K v
  note: stiffness
      | [NM/rad]
  note: K k
  note: LOAD
      | MOMENT INERTIA- gun
  note: 1/J L
  note: 1/J L
  note: stiffness
      | [NM/rad]
  note: T damp
  note: DAMPING
      | [NM/rad/sec]
  note: LOAD
      | MOMENT INERTIA
  note: K v
  note: T stif
  note: stiffness
      | [NM/rad]
  note: T damp
  note: DAMPING
      | [NM/rad/sec]
  note: LOAD
      | MOMENT INERTIA- turret
  note: K v
  note: 1/J L
  note: LOAD
      | MOMENT INERTIA- gun barrel
  note: amplifier
  current command traverse : Inport
  cant angle : Inport  Port=2
  Abs : Abs
  Add{1..2,4..5} (4 alike) : Sum
  Constant1 : Constant
  Cos : Trigonometry  Operator=cos
  Coulomb_Friction_Model : Subsystem
  Coulomb_Friction_Model1 : Subsystem
  Dead Zone1 : DeadZone  LowerValue=-0.07*10^-3  UpperValue=0.07*10^-3  ZeroCross=off
  Gain : Gain  Gain=1.84
  Gain1 : Gain  Gain=Kv2  mask{Kv2=0.1645}
      mask prompts: Kv2 "damping2"
  Gain10 : Gain  Gain=1/0.0065
  Gain13 : Gain  Gain=Kv2  mask{Kv2=0.015}
      mask prompts: Kv2 "damping2"
  Gain14 : Gain  Gain=0.6
  Gain15 : Gain  Gain=1/0.2189801
  Gain16 : Gain  Gain=Kk2  mask{Kk2=44.63119054}
      mask prompts: Kk2 "stifnes_2"
  Gain17 : Gain  Gain=Jl_inverse2  mask{Jl_inverse2=1/(3.649668334*10^-3)}
      mask prompts: Jl_inverse2 "inverse_moment_inertia2"
  Gain18 : Gain  Gain=328.0575777
  Gain2 : Gain  Gain=0.3525 /sqrt(3)
  Gain3 : Gain  Gain=1/0.0093
  Gain4 : Gain  Gain=1.7
  Gain5 : Gain  Gain=0.014
  Gain6 : Gain  Gain=1/(3.166864961*10^-3)
  Gain7 : Gain  Gain=Kk2  mask{Kk2=78.78413144}
      mask prompts: Kk2 "stifnes_2"
  Gain8 : Gain  Gain=Jl_inverse2  mask{Jl_inverse2=1/(3.649668334*10^-3)}
      mask prompts: Jl_inverse2 "inverse_moment_inertia2"
  Gain9 : Gain  Gain=4866/200
  Integrator{,4,6..7,9..11} (7 alike) : Integrator
  Integrator1 : Integrator  ZeroCross=off
  Integrator2 : Integrator  ExternalReset=rising  ShowStatePort=on  ZeroCross=off
  Integrator3 : Integrator  ZeroCross=off
  Integrator5 : Integrator  ExternalReset=rising  ShowStatePort=on  ZeroCross=off
  Integrator8 : Integrator  ZeroCross=off
  Product : Product
  Product1 : Product
  Scope : Scope
  Sign : Signum
  Sin : Trigonometry
  Sum1 : Sum  Inputs=-+|  SaturateOnIntegerOverflow=on
  Sum14 : Sum  Inputs=-+|-  SaturateOnIntegerOverflow=on
  Sum{2..3,6,9} (4 alike) : Sum  Inputs=|+-
  Sum4 : Sum  Inputs=-+|
  Sum5 : Sum  Inputs=-+|
  Sum7 : Sum  Inputs=-+|  SaturateOnIntegerOverflow=on
  Sum8 : Sum  Inputs=-+|  SaturateOnIntegerOverflow=on
  linearization backlash traverse : ManualSwitch  CurrentSetting=0
  linearization backlash1 az : ManualSwitch  CurrentSetting=0
  gun speed gyroscope : Outport
  motor speed tachometer : Outport  Port=2
  "gun angle gyroscope " : Outport  Port=3
  wires:
  Gain16/1 -> Integrator10/1
  Sum5/1 -> Coulomb_Friction_Model/1(Torque), Sum1/2
  Integrator7/1 -> Sum6/2
  Gain/1 -> Gain2/1
  Integrator9/1 -> Add1/1
  Gain3/1 -> Integrator5/1
  Gain13/1 -> Add4/2
  Add1/1 -> Sum4/2, Sum14/1
  Gain6/1 -> Integrator8/1
  Gain14/1 -> Product/1
  Gain2/1 -> Sum5/2
  Sum3/1 -> Gain7/1, Gain1/1
  Gain1/1 -> Add1/2
  Gain10/1 -> Integrator1/1
  Gain17/1 -> Integrator7/1
  Gain7/1 -> Integrator9/1
  Integrator8/1 -> Sum2/2  "velocity_feedback"
  Integrator3/1 -> gun speed gyroscope/1, Integrator4/1, Sum3/2, Integrator11/1, Sum6/1
  Sum2/1 -> Integrator6/1, Gain5/1
  Sum4/1 -> Gain8/1
  Add4/1 -> Sum4/1, Gain17/1
  Integrator10/1 -> Add4/1
  Integrator2/1 -> Coulomb_Friction_Model1/2(velocity), Sum3/1, Sum9/2  "velocity_feedback"
  Sum9/1 -> Gain14/1, Integrator/1
  Sum6/1 -> Gain16/1, Gain13/1
  Gain15/1 -> Integrator2/1
  Sum7/1 -> Gain10/1
  Add2/1 -> Gain6/1, Sum7/1
  Sum1/1 -> Sum7/2, Gain3/1
  Integrator5/1 -> Coulomb_Friction_Model/2(velocity), Sum9/1  "velocity_feedback"
  Add5/1 -> Sum5/1, Sum14/2
  Gain8/1 -> Integrator3/1
  Integrator1/1 -> motor speed tachometer/1, Sum2/1  "velocity_feedback"
  current command traverse/1 -> Gain/1
  Sign/1 -> linearization backlash traverse/2
  Abs/1 -> Sign/1
  linearization backlash traverse/1 -> Product/2
  Constant1/1 -> linearization backlash traverse/1
  Product/1 -> Add5/2
  Dead Zone1/1 -> linearization backlash1 az/2
  Integrator/1 -> linearization backlash1 az/1, Dead Zone1/1
  linearization backlash1 az/1 -> Abs/1, Gain18/1
  Gain18/1 -> Add5/1
  Gain4/1 -> Add2/1
  Gain5/1 -> Add2/2
  Integrator6/1 -> Gain4/1
  Coulomb_Friction_Model/1(Friction_Torque) -> Sum1/1
  Integrator5/State -> Coulomb_Friction_Model/3(velocity state)
  Coulomb_Friction_Model/2(reset velocity) -> Integrator5/2
  Sum8/1 -> Gain15/1
  Sum14/1 -> Coulomb_Friction_Model1/1(Torque), Sum8/2
  Coulomb_Friction_Model1/1(Friction_Torque) -> Sum8/1
  Integrator2/State -> Coulomb_Friction_Model1/3(velocity state)
  Coulomb_Friction_Model1/2(reset velocity) -> Integrator2/2
  Integrator11/1 -> "gun angle gyroscope "/1
  Sin/1 -> Gain9/1
  Integrator4/1 -> Sin/1
  cant angle/1 -> Cos/1
  Gain9/1 -> Product1/1
  Cos/1 -> Product1/2
  Product1/1 -> Sum14/3

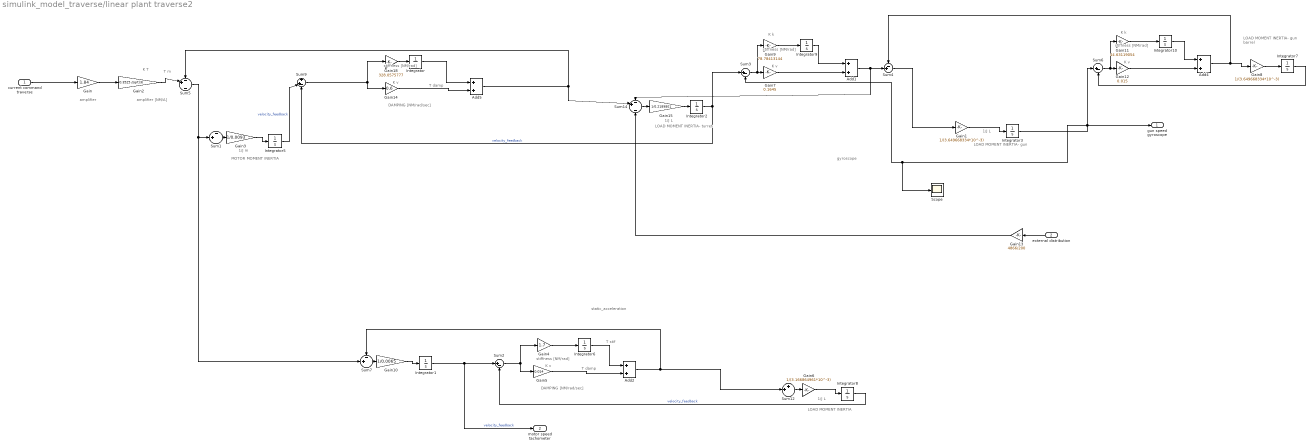
== system simulink_model_traverse/linear plant traverse2 ==
  note: gyroscope
  note: K v
  note: T m
  note: stiffness
      | [NM/rad]
  note: K T
  note: K k
  note: MOTOR
      | MOMENT INERTIA
  note: amplifier
      | [NM/A]
  note: 1/J m
  note: K v
  note: stiffness
      | [NM/rad]
  note: K k
  note: static_acceleration
  note: LOAD
      | MOMENT INERTIA- gun
  note: 1/J L
  note: 1/J L
  note: stiffness
      | [NM/rad]
  note: T damp
  note: DAMPING
      | [NM/rad/sec]
  note: LOAD
      | MOMENT INERTIA
  note: K v
  note: T stif
  note: stiffness
      | [NM/rad]
  note: T damp
  note: DAMPING
      | [NM/rad/sec]
  note: LOAD
      | MOMENT INERTIA- turret
  note: K v
  note: 1/J L
  note: LOAD
      | MOMENT INERTIA- gun barrel
  note: amplifier
  current command traverse : Inport
  external distribution : Inport  Port=2
  Add{1..2,4..5} (4 alike) : Sum
  Gain : Gain  Gain=1.84
  Gain1 : Gain  Gain=1/(3.649668334*10^-3)
  Gain10 : Gain  Gain=1/0.0065
  Gain11 : Gain  Gain=44.63119054
  Gain12 : Gain  Gain=0.015
  Gain13 : Gain  Gain=4866/200
  Gain14 : Gain  Gain=0.6
  Gain15 : Gain  Gain=1/0.2189801
  Gain18 : Gain  Gain=328.0575777
  Gain2 : Gain  Gain=0.3525 /sqrt(3)
  Gain3 : Gain  Gain=1/0.0093
  Gain4 : Gain  Gain=1.7
  Gain5 : Gain  Gain=0.014
  Gain6 : Gain  Gain=1/(3.166864961*10^-3)
  Gain7 : Gain  Gain=0.1645
  Gain8 : Gain  Gain=1/(3.649668334*10^-3)
  Gain9 : Gain  Gain=78.78413144
  Integrator{,6..7,9..10} (5 alike) : Integrator
  Integrator{1..3,5,8} (5 alike) : Integrator  ZeroCross=off
  Scope : Scope
  Sum1 : Sum  Inputs=-+|  SaturateOnIntegerOverflow=on
  Sum12 : Sum  Inputs=++|  SaturateOnIntegerOverflow=on
  Sum14 : Sum  Inputs=-+|-  SaturateOnIntegerOverflow=on
  Sum2 : Sum  Inputs=|+-
  Sum3 : Sum  Inputs=|+-
  Sum4 : Sum  Inputs=-+|
  Sum5 : Sum  Inputs=-+|-
  Sum6 : Sum  Inputs=|+-
  Sum7 : Sum  Inputs=-+|  SaturateOnIntegerOverflow=on
  Sum9 : Sum  Inputs=+|+-
  gun speed gyroscope : Outport
  motor speed tachometer : Outport  Port=2
  wires:
  Gain11/1 -> Integrator10/1
  Sum5/1 -> Sum7/2, Sum1/2
  Integrator7/1 -> Sum6/2
  Gain/1 -> Gain2/1
  Integrator9/1 -> Add1/1
  Gain18/1 -> Integrator/1
  Gain3/1 -> Integrator5/1
  Gain12/1 -> Add4/2
  Add1/1 -> Sum14/1, Sum4/2
  Gain6/1 -> Integrator8/1
  Gain14/1 -> Add5/2
  Gain2/1 -> Sum5/2
  Integrator/1 -> Add5/1
  Sum3/1 -> Gain7/1, Gain9/1
  Gain7/1 -> Add1/2
  Gain10/1 -> Integrator1/1
  Gain8/1 -> Integrator7/1
  Gain9/1 -> Integrator9/1
  Integrator8/1 -> Sum2/2  "velocity_feedback"
  Integrator3/1 -> gun speed gyroscope/1, Scope/1, Sum3/2, Sum6/1
  Sum2/1 -> Gain5/1, Gain4/1
  Sum4/1 -> Gain1/1
  Add4/1 -> Gain8/1, Sum4/1
  Integrator10/1 -> Add4/1
  Add2/1 -> Sum7/1, Sum12/2
  Integrator6/1 -> Add2/1
  Integrator2/1 -> Sum9/3, Sum3/1  "velocity_feedback"
  Sum9/1 -> Gain18/1, Gain14/1
  Sum6/1 -> Gain12/1, Gain11/1
  Sum14/1 -> Gain15/1
  Gain15/1 -> Integrator2/1
  Gain5/1 -> Add2/2
  Sum7/1 -> Gain10/1
  Sum12/1 -> Gain6/1
  Sum1/1 -> Gain3/1
  Add5/1 -> Sum14/2, Sum5/1
  Gain4/1 -> Integrator6/1
  Gain1/1 -> Integrator3/1
  Integrator1/1 -> motor speed tachometer/1, Sum2/1  "velocity_feedback"
  current command traverse/1 -> Gain/1
  Integrator5/1 -> Sum9/2  "velocity_feedback"
  ? -> ?
  external distribution/1 -> Gain13/1
  Gain13/1 -> Sum14/3

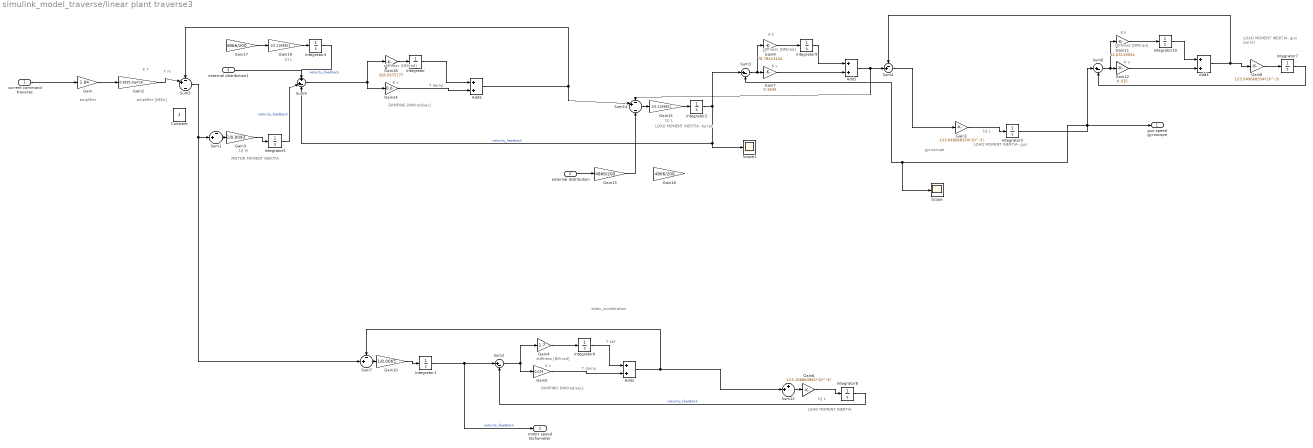
== system simulink_model_traverse/linear plant traverse3 ==
  note: gyroscope
  note: K v
  note: T m
  note: stiffness
      | [NM/rad]
  note: K T
  note: K k
  note: MOTOR
      | MOMENT INERTIA
  note: amplifier
      | [NM/A]
  note: 1/J m
  note: K v
  note: stiffness
      | [NM/rad]
  note: K k
  note: static_acceleration
  note: LOAD
      | MOMENT INERTIA- gun
  note: 1/J L
  note: 1/J L
  note: stiffness
      | [NM/rad]
  note: T damp
  note: DAMPING
      | [NM/rad/sec]
  note: LOAD
      | MOMENT INERTIA
  note: K v
  note: T stif
  note: stiffness
      | [NM/rad]
  note: T damp
  note: DAMPING
      | [NM/rad/sec]
  note: LOAD
      | MOMENT INERTIA- turret
  note: K v
  note: 1/J L
  note: LOAD
      | MOMENT INERTIA- gun barrel
  note: amplifier
  note: 1/J L
  current command traverse : Inport
  external distribution : Inport  Port=2
  external distribution1 : Inport  Port=3
  Add{1..2,4..5} (4 alike) : Sum
  Constant : Constant
  Gain : Gain  Gain=1.84
  Gain1 : Gain  Gain=1/(3.649668334*10^-3)
  Gain10 : Gain  Gain=1/0.0065
  Gain11 : Gain  Gain=44.63119054
  Gain12 : Gain  Gain=0.015
  Gain13 : Gain  Gain=4866/200
  Gain14 : Gain  Gain=0.6
  Gain15 : Gain  Gain=1/0.2189801
  Gain16 : Gain  Gain=4866/200
  Gain17 : Gain  Gain=4866/200
  Gain18 : Gain  Gain=328.0575777
  Gain19 : Gain  Gain=1/0.2189801
  Gain2 : Gain  Gain=0.3525 /sqrt(3)
  Gain3 : Gain  Gain=1/0.0093
  Gain4 : Gain  Gain=1.7
  Gain5 : Gain  Gain=0.014
  Gain6 : Gain  Gain=1/(3.166864961*10^-3)
  Gain7 : Gain  Gain=0.1645
  Gain8 : Gain  Gain=1/(3.649668334*10^-3)
  Gain9 : Gain  Gain=78.78413144
  Integrator{,6..7,9..10} (5 alike) : Integrator
  Integrator{1..5,8} (6 alike) : Integrator  ZeroCross=off
  Scope : Scope
  Scope1 : Scope
  Sum1 : Sum  Inputs=-+|  SaturateOnIntegerOverflow=on
  Sum12 : Sum  Inputs=++|  SaturateOnIntegerOverflow=on
  Sum14 : Sum  Inputs=-+|-  SaturateOnIntegerOverflow=on
  Sum2 : Sum  Inputs=|+-
  Sum3 : Sum  Inputs=|+-
  Sum4 : Sum  Inputs=-+|
  Sum5 : Sum  Inputs=-+|-
  Sum6 : Sum  Inputs=|+-
  Sum7 : Sum  Inputs=-+|  SaturateOnIntegerOverflow=on
  Sum9 : Sum  Inputs=+|+-
  gun speed gyroscope : Outport
  motor speed tachometer : Outport  Port=2
  wires:
  Gain11/1 -> Integrator10/1
  Sum5/1 -> Sum7/2, Sum1/2
  Integrator7/1 -> Sum6/2
  Gain/1 -> Gain2/1
  Integrator9/1 -> Add1/1
  Gain18/1 -> Integrator/1
  Gain3/1 -> Integrator5/1
  Gain12/1 -> Add4/2
  Add1/1 -> Sum14/1, Sum4/2
  Gain6/1 -> Integrator8/1
  Gain14/1 -> Add5/2
  Gain2/1 -> Sum5/2
  Integrator/1 -> Add5/1
  Sum3/1 -> Gain7/1, Gain9/1
  Gain7/1 -> Add1/2
  Gain10/1 -> Integrator1/1
  Gain8/1 -> Integrator7/1
  Gain9/1 -> Integrator9/1
  Integrator8/1 -> Sum2/2  "velocity_feedback"
  Integrator3/1 -> gun speed gyroscope/1, Scope/1, Sum3/2, Sum6/1
  Sum2/1 -> Gain5/1, Gain4/1
  Sum4/1 -> Gain1/1
  Add4/1 -> Gain8/1, Sum4/1
  Integrator10/1 -> Add4/1
  Add2/1 -> Sum7/1, Sum12/2
  Integrator6/1 -> Add2/1
  Integrator2/1 -> Scope1/1, Sum9/3, Sum3/1  "velocity_feedback"
  Sum9/1 -> Gain18/1, Gain14/1
  Sum6/1 -> Gain12/1, Gain11/1
  Sum14/1 -> Gain15/1
  Gain15/1 -> Integrator2/1
  Gain5/1 -> Add2/2
  Sum7/1 -> Gain10/1
  Sum12/1 -> Gain6/1
  Sum1/1 -> Gain3/1
  Add5/1 -> Sum14/2, Sum5/1
  Gain4/1 -> Integrator6/1
  Gain1/1 -> Integrator3/1
  Integrator1/1 -> motor speed tachometer/1, Sum2/1  "velocity_feedback"
  current command traverse/1 -> Gain/1
  Integrator5/1 -> Sum9/2  "velocity_feedback"
  Gain13/1 -> Sum14/3
  external distribution/1 -> Gain13/1
  Gain19/1 -> Integrator4/1
  Gain17/1 -> Gain19/1
  Integrator4/1 -> ?  "velocity_feedback"
  external distribution1/1 -> Sum9/1

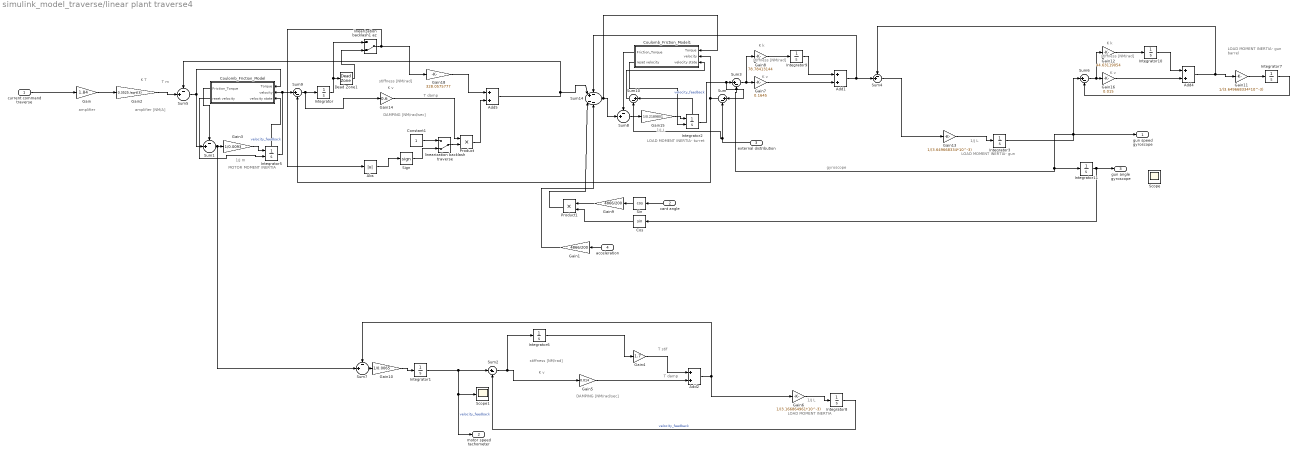
== system simulink_model_traverse/linear plant traverse4 ==
  note: gyroscope
  note: K v
  note: T m
  note: stiffness
      | [NM/rad]
  note: K T
  note: K k
  note: MOTOR
      | MOMENT INERTIA
  note: amplifier
      | [NM/A]
  note: 1/J m
  note: K v
  note: stiffness
      | [NM/rad]
  note: K k
  note: LOAD
      | MOMENT INERTIA- gun
  note: 1/J L
  note: 1/J L
  note: stiffness
      | [NM/rad]
  note: T damp
  note: DAMPING
      | [NM/rad/sec]
  note: LOAD
      | MOMENT INERTIA
  note: K v
  note: T stif
  note: stiffness
      | [NM/rad]
  note: T damp
  note: DAMPING
      | [NM/rad/sec]
  note: LOAD
      | MOMENT INERTIA- turret
  note: K v
  note: 1/J L
  note: LOAD
      | MOMENT INERTIA- gun barrel
  note: amplifier
  current command traverse : Inport
  cant angle : Inport  Port=2
  external distribution : Inport  Port=3
  acceleration : Inport  Port=4
  Abs : Abs
  Add{1..2,4..5} (4 alike) : Sum
  Constant1 : Constant
  Cos : Trigonometry
  Coulomb_Friction_Model : Subsystem
  Coulomb_Friction_Model1 : Subsystem
  Dead Zone1 : DeadZone  LowerValue=-0.07*10^-3  UpperValue=0.07*10^-3  ZeroCross=off
  Gain : Gain  Gain=1.84
  Gain1 : Gain  Gain=4866/200
  Gain10 : Gain  Gain=1/0.0065
  Gain11 : Gain  Gain=1/(3.649668334*10^-3)
  Gain12 : Gain  Gain=44.63119054
  Gain13 : Gain  Gain=1/(3.649668334*10^-3)
  Gain14 : Gain  Gain=0.6
  Gain15 : Gain  Gain=1/0.2189801
  Gain16 : Gain  Gain=0.015
  Gain18 : Gain  Gain=328.0575777
  Gain2 : Gain  Gain=0.3525 /sqrt(3)
  Gain3 : Gain  Gain=1/0.0093
  Gain4 : Gain  Gain=1.7
  Gain5 : Gain  Gain=0.014
  Gain6 : Gain  Gain=1/(3.166864961*10^-3)
  Gain7 : Gain  Gain=0.1645
  Gain8 : Gain  Gain=78.78413144
  Gain9 : Gain  Gain=4866/200
  Integrator{,6..7,9..11} (6 alike) : Integrator
  Integrator1 : Integrator  ZeroCross=off
  Integrator2 : Integrator  ExternalReset=rising  ShowStatePort=on  ZeroCross=off
  Integrator3 : Integrator  ZeroCross=off
  Integrator5 : Integrator  ExternalReset=rising  ShowStatePort=on  ZeroCross=off
  Integrator8 : Integrator  ZeroCross=off
  Product : Product
  Product1 : Product
  Scope : Scope
  Scope1 : Scope
  Sign : Signum
  Sin : Trigonometry  Operator=cos
  Sum{,2..3,6,9..10} (6 alike) : Sum  Inputs=|+-
  Sum1 : Sum  Inputs=-+|  SaturateOnIntegerOverflow=on
  Sum14 : Sum  Inputs=-+|--  SaturateOnIntegerOverflow=on
  Sum4 : Sum  Inputs=-+|
  Sum5 : Sum  Inputs=-+|
  Sum7 : Sum  Inputs=-+|  SaturateOnIntegerOverflow=on
  Sum8 : Sum  Inputs=-+|  SaturateOnIntegerOverflow=on
  linearization backlash traverse : ManualSwitch  CurrentSetting=0
  linearization backlash1 az : ManualSwitch  CurrentSetting=0
  gun speed gyroscope : Outport
  motor speed tachometer : Outport  Port=2
  "gun angle gyroscope " : Outport  Port=3
  wires:
  Gain12/1 -> Integrator10/1
  Sum5/1 -> Coulomb_Friction_Model/1(Torque), Sum1/2
  Integrator7/1 -> Sum6/2
  Gain/1 -> Gain2/1
  Integrator9/1 -> Add1/1
  Gain3/1 -> Integrator5/1
  Gain16/1 -> Add4/2
  Add1/1 -> Sum4/2, Sum14/1
  Gain6/1 -> Integrator8/1
  Gain14/1 -> Product/1
  Gain2/1 -> Sum5/2
  Sum3/1 -> Gain7/1, Gain8/1
  Gain7/1 -> Add1/2
  Gain10/1 -> Integrator1/1
  Gain11/1 -> Integrator7/1
  Gain8/1 -> Integrator9/1
  Integrator8/1 -> Sum2/2  "velocity_feedback"
  Integrator3/1 -> gun speed gyroscope/1, Sum3/2, Integrator11/1, Sum6/1
  Sum2/1 -> Integrator6/1, Gain5/1
  Sum4/1 -> Gain13/1
  Add4/1 -> Gain11/1, Sum4/1
  Integrator10/1 -> Add4/1
  Integrator2/1 -> Sum/1, Sum3/1  "velocity_feedback"
  Sum9/1 -> Gain14/1, Integrator/1
  Sum6/1 -> Gain16/1, Gain12/1
  Gain15/1 -> Integrator2/1
  Sum7/1 -> Gain10/1
  Add2/1 -> Gain6/1, Sum7/1
  Sum1/1 -> Sum7/2, Gain3/1
  Integrator5/1 -> Coulomb_Friction_Model/2(velocity), Sum9/1  "velocity_feedback"
  Add5/1 -> Sum5/1, Sum14/2
  Gain13/1 -> Integrator3/1
  Integrator1/1 -> motor speed tachometer/1, Scope1/1, Sum2/1  "velocity_feedback"
  current command traverse/1 -> Gain/1
  Sign/1 -> linearization backlash traverse/2
  Abs/1 -> Sign/1
  linearization backlash traverse/1 -> Product/2
  Constant1/1 -> linearization backlash traverse/1
  Product/1 -> Add5/2
  Dead Zone1/1 -> linearization backlash1 az/2
  Integrator/1 -> linearization backlash1 az/1, Dead Zone1/1
  linearization backlash1 az/1 -> Abs/1, Gain18/1
  Gain18/1 -> Add5/1
  Gain4/1 -> Add2/1
  Gain5/1 -> Add2/2
  Integrator6/1 -> Gain4/1
  Coulomb_Friction_Model/1(Friction_Torque) -> Sum1/1
  Coulomb_Friction_Model/2(reset velocity) -> Integrator5/2
  Sum8/1 -> Gain15/1
  Sum14/1 -> Coulomb_Friction_Model1/1(Torque), Sum8/2
  Coulomb_Friction_Model1/1(Friction_Torque) -> Sum8/1
  Coulomb_Friction_Model1/2(reset velocity) -> Integrator2/2
  Integrator11/1 -> Cos/1, "gun angle gyroscope "/1
  Sin/1 -> Gain9/1
  Gain9/1 -> Product1/1
  cant angle/1 -> Sin/1
  Sum/1 -> Coulomb_Friction_Model1/2(velocity), Sum9/2
  Sum10/1 -> Coulomb_Friction_Model1/3(velocity state)
  external distribution/1 -> Sum10/2, Sum/2
  Integrator5/State -> Coulomb_Friction_Model/3(velocity state)
  Integrator2/State -> Sum10/1
  Cos/1 -> Product1/2
  Product1/1 -> Sum14/3
  acceleration/1 -> Gain1/1
  Gain1/1 -> Sum14/4

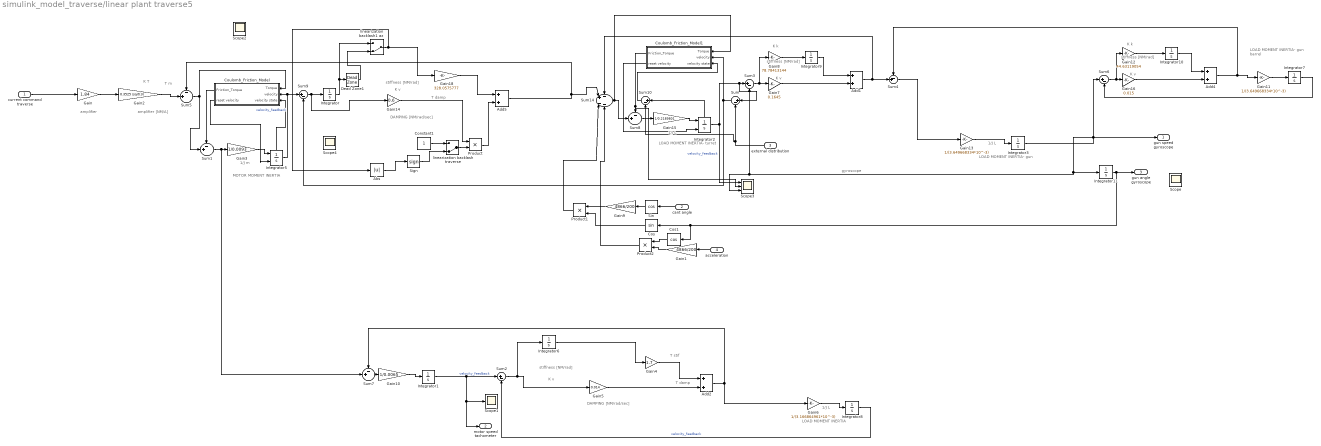
== system simulink_model_traverse/linear plant traverse5 ==
  note: gyroscope
  note: K v
  note: T m
  note: stiffness
      | [NM/rad]
  note: K T
  note: K k
  note: MOTOR
      | MOMENT INERTIA
  note: amplifier
      | [NM/A]
  note: 1/J m
  note: K v
  note: stiffness
      | [NM/rad]
  note: K k
  note: LOAD
      | MOMENT INERTIA- gun
  note: 1/J L
  note: 1/J L
  note: stiffness
      | [NM/rad]
  note: T damp
  note: DAMPING
      | [NM/rad/sec]
  note: LOAD
      | MOMENT INERTIA
  note: K v
  note: T stif
  note: stiffness
      | [NM/rad]
  note: T damp
  note: DAMPING
      | [NM/rad/sec]
  note: LOAD
      | MOMENT INERTIA- turret
  note: K v
  note: 1/J L
  note: LOAD
      | MOMENT INERTIA- gun barrel
  note: amplifier
  current command traverse : Inport
  cant angle : Inport  Port=2
  external distribution : Inport  Port=3
  acceleration : Inport  Port=4
  Abs : Abs
  Add{1..2,4..5} (4 alike) : Sum
  Constant1 : Constant
  Cos : Trigonometry
  Cos1 : Trigonometry  Operator=cos
  Coulomb_Friction_Model : Subsystem
  Coulomb_Friction_Model1 : Subsystem
  Dead Zone1 : DeadZone  LowerValue=-0.07*10^-3  UpperValue=0.07*10^-3  ZeroCross=off
  Gain : Gain  Gain=1.84
  Gain1 : Gain  Gain=4866/200
  Gain10 : Gain  Gain=1/0.0065
  Gain11 : Gain  Gain=1/(3.649668334*10^-3)
  Gain12 : Gain  Gain=44.63119054
  Gain13 : Gain  Gain=1/(3.649668334*10^-3)
  Gain14 : Gain  Gain=0.6
  Gain15 : Gain  Gain=1/0.2189801
  Gain16 : Gain  Gain=0.015
  Gain18 : Gain  Gain=328.0575777
  Gain2 : Gain  Gain=0.3525 /sqrt(3)
  Gain3 : Gain  Gain=1/0.0093
  Gain4 : Gain  Gain=1.7
  Gain5 : Gain  Gain=0.014
  Gain6 : Gain  Gain=1/(3.166864961*10^-3)
  Gain7 : Gain  Gain=0.1645
  Gain8 : Gain  Gain=78.78413144
  Gain9 : Gain  Gain=4866/200
  Integrator{,6..7,9..11} (6 alike) : Integrator
  Integrator1 : Integrator  ZeroCross=off
  Integrator2 : Integrator  ExternalReset=rising  ShowStatePort=on  ZeroCross=off
  Integrator3 : Integrator  ZeroCross=off
  Integrator5 : Integrator  ExternalReset=rising  ShowStatePort=on  ZeroCross=off
  Integrator8 : Integrator  ZeroCross=off
  Product : Product
  Product1 : Product
  Product2 : Product
  Scope{,1..2,4} (4 alike) : Scope
  Scope3 : Scope  NumInputPorts=3
  Sign : Signum
  Sin : Trigonometry  Operator=cos
  Sum{,2..3,6,9..10} (6 alike) : Sum  Inputs=|+-
  Sum1 : Sum  Inputs=-+|  SaturateOnIntegerOverflow=on
  Sum14 : Sum  Inputs=-+|--  SaturateOnIntegerOverflow=on
  Sum4 : Sum  Inputs=-+|
  Sum5 : Sum  Inputs=-+|
  Sum7 : Sum  Inputs=-+|  SaturateOnIntegerOverflow=on
  Sum8 : Sum  Inputs=-+|  SaturateOnIntegerOverflow=on
  linearization backlash traverse : ManualSwitch  CurrentSetting=0
  linearization backlash1 az : ManualSwitch  CurrentSetting=0
  gun speed gyroscope : Outport
  motor speed tachometer : Outport  Port=2
  "gun angle gyroscope " : Outport  Port=3
  wires:
  Gain12/1 -> Integrator10/1
  Sum5/1 -> Coulomb_Friction_Model/1(Torque), Sum1/2
  Integrator7/1 -> Sum6/2
  Gain/1 -> Gain2/1
  Integrator9/1 -> Add1/1
  Gain3/1 -> Integrator5/1
  Gain16/1 -> Add4/2
  Add1/1 -> Sum4/2, Sum14/1
  Gain6/1 -> Integrator8/1
  Gain14/1 -> Product/1
  Gain2/1 -> Sum5/2
  Sum3/1 -> Gain7/1, Gain8/1
  Gain7/1 -> Add1/2
  Gain10/1 -> Integrator1/1
  Gain11/1 -> Integrator7/1
  Gain8/1 -> Integrator9/1
  Integrator8/1 -> Sum2/2  "velocity_feedback"
  Integrator3/1 -> gun speed gyroscope/1, Scope3/3, Sum3/2, Integrator11/1, Sum6/1
  Sum2/1 -> Integrator6/1, Gain5/1
  Sum4/1 -> Gain13/1
  Add4/1 -> Gain11/1, Sum4/1
  Integrator10/1 -> Add4/1
  Integrator2/1 -> Scope3/1, Sum/1, Sum3/1  "velocity_feedback"
  Sum9/1 -> Gain14/1, Integrator/1
  Sum6/1 -> Gain16/1, Gain12/1
  Gain15/1 -> Integrator2/1
  Sum7/1 -> Gain10/1
  Add2/1 -> Gain6/1, Sum7/1
  Sum1/1 -> Sum7/2, Gain3/1
  Integrator5/1 -> Coulomb_Friction_Model/2(velocity), Sum9/1  "velocity_feedback"
  Add5/1 -> Sum5/1, Sum14/2
  Gain13/1 -> Integrator3/1
  Integrator1/1 -> motor speed tachometer/1, Scope1/1, Sum2/1  "velocity_feedback"
  current command traverse/1 -> Gain/1
  Sign/1 -> linearization backlash traverse/2
  Abs/1 -> Sign/1
  linearization backlash traverse/1 -> Product/2
  Constant1/1 -> linearization backlash traverse/1
  Product/1 -> Add5/2
  Dead Zone1/1 -> linearization backlash1 az/2
  Integrator/1 -> linearization backlash1 az/1, Dead Zone1/1
  linearization backlash1 az/1 -> Abs/1, Gain18/1
  Gain18/1 -> Add5/1
  Gain4/1 -> Add2/1
  Gain5/1 -> Add2/2
  Integrator6/1 -> Gain4/1
  Sum8/1 -> Gain15/1
  Sum14/1 -> Sum8/2, Coulomb_Friction_Model1/1(Torque)
  Coulomb_Friction_Model1/1(Friction_Torque) -> Scope3/2, Sum8/1
  Integrator11/1 -> Cos1/1, Cos/1, "gun angle gyroscope "/1
  Sin/1 -> Gain9/1
  Gain9/1 -> Product1/1
  cant angle/1 -> Sin/1
  Sum/1 -> Coulomb_Friction_Model1/2(velocity), Sum9/2
  Sum10/1 -> Coulomb_Friction_Model1/3(velocity state)
  external distribution/1 -> Sum10/2, Sum/2
  Integrator2/State -> Sum10/1
  Cos/1 -> Product1/2
  acceleration/1 -> Gain1/1
  Product1/1 -> Sum14/3
  Coulomb_Friction_Model1/2(reset velocity) -> Integrator2/2
  Gain1/1 -> Product2/2
  Cos1/1 -> Product2/1
  Product2/1 -> Sum14/4
  Coulomb_Friction_Model/1(Friction_Torque) -> Sum1/1
  Coulomb_Friction_Model/2(reset velocity) -> Integrator5/2
  Integrator5/State -> Coulomb_Friction_Model/3(velocity state)

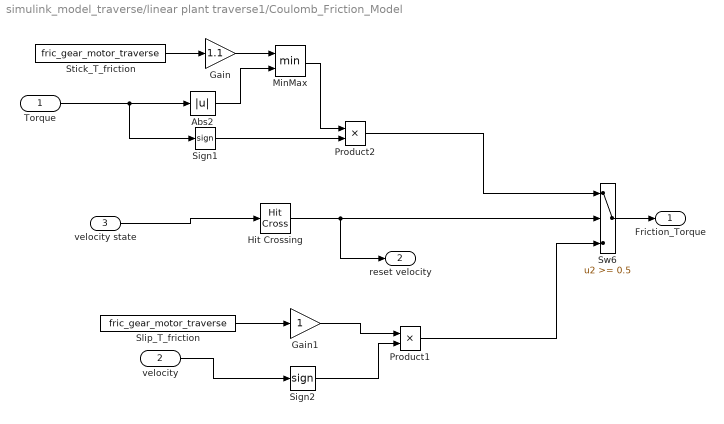
== system simulink_model_traverse/linear plant traverse1/Coulomb_Friction_Model ==
  Torque : Inport
  velocity : Inport  Port=2
  velocity state : Inport  Port=3
  Abs2 : Abs  ZeroCross=off
  Gain : Gain  Gain=1.1
  Gain1 : Gain
  Hit Crossing : HitCross  ZeroCross=off
  MinMax : MinMax  Inputs=2
  Product1 : Product  RndMeth=Zero
  Product2 : Product  RndMeth=Zero
  Sign1 : Signum  ZeroCross=off
  Sign2 : Signum  ZeroCross=off
  Slip_T_friction : Constant  Value=fric_gear_motor_traverse
  Stick_T_friction : Constant  Value=fric_gear_motor_traverse
  Sw6 : Switch  Threshold=0.5  ZeroCross=off  SaturateOnIntegerOverflow=on  InputSameDT=on
  Friction_Torque : Outport
  reset velocity : Outport  Port=2
  wires:
  Torque/1 -> Sign1/1, Abs2/1
  Sw6/1 -> Friction_Torque/1
  Hit Crossing/1 -> reset velocity/1, Sw6/2
  Abs2/1 -> MinMax/2
  MinMax/1 -> Product2/1
  Product2/1 -> Sw6/1
  Product1/1 -> Sw6/3
  Sign2/1 -> Product1/2
  velocity/1 -> Sign2/1
  Sign1/1 -> Product2/2
  velocity state/1 -> Hit Crossing/1
  Stick_T_friction/1 -> Gain/1
  Gain/1 -> MinMax/1
  Slip_T_friction/1 -> Gain1/1
  Gain1/1 -> Product1/1

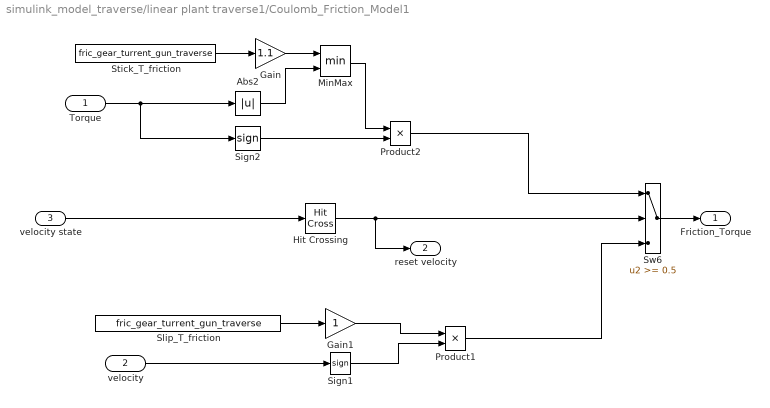
== system simulink_model_traverse/linear plant traverse1/Coulomb_Friction_Model1 ==
  Torque : Inport
  velocity : Inport  Port=2
  velocity state : Inport  Port=3
  Abs2 : Abs  ZeroCross=off
  Gain : Gain  Gain=1.1
  Gain1 : Gain
  Hit Crossing : HitCross  ZeroCross=off
  MinMax : MinMax  Inputs=2
  Product1 : Product  RndMeth=Zero
  Product2 : Product  RndMeth=Zero
  Sign1 : Signum  ZeroCross=off
  Sign2 : Signum  ZeroCross=off
  Slip_T_friction : Constant  Value=fric_gear_turrent_gun_traverse  SampleTime=0
  Stick_T_friction : Constant  Value=fric_gear_turrent_gun_traverse  SampleTime=0
  Sw6 : Switch  Threshold=0.5  ZeroCross=off  SaturateOnIntegerOverflow=on  InputSameDT=on
  Friction_Torque : Outport
  reset velocity : Outport  Port=2
  wires:
  Torque/1 -> Sign2/1, Abs2/1
  Sw6/1 -> Friction_Torque/1
  Hit Crossing/1 -> reset velocity/1, Sw6/2
  Abs2/1 -> MinMax/2
  MinMax/1 -> Product2/1
  Product2/1 -> Sw6/1
  Product1/1 -> Sw6/3
  velocity/1 -> Sign1/1
  Sign1/1 -> Product1/2
  Sign2/1 -> Product2/2
  velocity state/1 -> Hit Crossing/1
  Gain/1 -> MinMax/1
  Stick_T_friction/1 -> Gain/1
  Slip_T_friction/1 -> Gain1/1
  Gain1/1 -> Product1/1

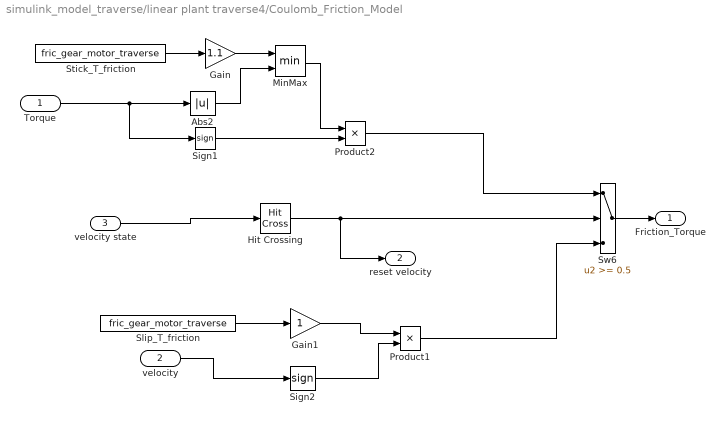
== system simulink_model_traverse/linear plant traverse4/Coulomb_Friction_Model ==
  Torque : Inport
  velocity : Inport  Port=2
  velocity state : Inport  Port=3
  Abs2 : Abs  ZeroCross=off
  Gain : Gain  Gain=1.1
  Gain1 : Gain
  Hit Crossing : HitCross  ZeroCross=off
  MinMax : MinMax  Inputs=2
  Product1 : Product  RndMeth=Zero
  Product2 : Product  RndMeth=Zero
  Sign1 : Signum  ZeroCross=off
  Sign2 : Signum  ZeroCross=off
  Slip_T_friction : Constant  Value=fric_gear_motor_traverse
  Stick_T_friction : Constant  Value=fric_gear_motor_traverse
  Sw6 : Switch  Threshold=0.5  ZeroCross=off  SaturateOnIntegerOverflow=on  InputSameDT=on
  Friction_Torque : Outport
  reset velocity : Outport  Port=2
  wires:
  Torque/1 -> Sign1/1, Abs2/1
  Sw6/1 -> Friction_Torque/1
  Hit Crossing/1 -> reset velocity/1, Sw6/2
  Abs2/1 -> MinMax/2
  MinMax/1 -> Product2/1
  Product2/1 -> Sw6/1
  Product1/1 -> Sw6/3
  Sign2/1 -> Product1/2
  velocity/1 -> Sign2/1
  Sign1/1 -> Product2/2
  velocity state/1 -> Hit Crossing/1
  Stick_T_friction/1 -> Gain/1
  Gain/1 -> MinMax/1
  Slip_T_friction/1 -> Gain1/1
  Gain1/1 -> Product1/1
